simulink model "MSDR_v1"  (R2018a)
settings: Solver=ode23tb  StartTime=0.0  StopTime=50000  RelTol=1e-3
values from neighbouring files (symbols this model uses):
  a_f = -3.22E-5    (= -3.22e-05)    [MSDR_parameters.m]
  a_g = +2.35E-5    (= 2.35e-05)    [MSDR_parameters.m]
  beta = [0.000223, 0.001457, 0.001307, 0.002628, 0.000766, 0.000280]    [MSDR_parameters.m]
  beta_t = sum(beta)    [MSDR_parameters.m]
  Cp_s_shx = 1549.12e-6    (= 0.00154912)    [MSDR_parameters.m]
  Cst = 10    [MSDR_parameters.m]
  dLb = 0    [MSDR_parameters.m]
  dLs = 0    [MSDR_parameters.m]
  dLsc = 0    [MSDR_parameters.m]
  gamma_I = 5.1135e-2    (= 0.051135)    [MSDR_parameters.m]
  gamma_Xe = 1.1628e-2    (= 0.011628)    [MSDR_parameters.m]
  hA_fg = [h_fg*A_fg/2, h_fg*A_fg/2]    [MSDR_parameters.m]
  hA_p_phx1 = h_p_phx*A_p_phx    [MSDR_parameters.m]
  hA_p_phx2 = h_p_phx*A_p_phx    [MSDR_parameters.m]
  hA_p_phx3 = h_p_phx*A_p_phx    [MSDR_parameters.m]
  hA_p_phx4 = h_p_phx*A_p_phx    [MSDR_parameters.m]
  hA_p_phx5 = h_p_phx*A_p_phx    [MSDR_parameters.m]
  hA_p_phx6 = h_p_phx*A_p_phx    [MSDR_parameters.m]
  hA_p_shx1 = h_p_shx*A_p_shx    [MSDR_parameters.m]
  hA_p_shx2 = h_p_shx*A_p_shx    [MSDR_parameters.m]
  hA_p_shx3 = h_p_shx*A_p_shx    [MSDR_parameters.m]
  hA_p_shx4 = h_p_shx*A_p_shx    [MSDR_parameters.m]
  hA_p_shx5 = h_p_shx*A_p_shx    [MSDR_parameters.m]
  hA_p_shx6 = h_p_shx*A_p_shx    [MSDR_parameters.m]
  hA_s_phx1 = h_s_phx*A_s_phx    [MSDR_parameters.m]
  hA_s_phx2 = h_s_phx*A_s_phx    [MSDR_parameters.m]
  hA_s_phx3 = h_s_phx*A_s_phx    [MSDR_parameters.m]
  hA_s_phx4 = h_s_phx*A_s_phx    [MSDR_parameters.m]
  hA_s_phx5 = h_s_phx*A_s_phx    [MSDR_parameters.m]
  hA_s_phx6 = h_s_phx*A_s_phx    [MSDR_parameters.m]
  hA_s_shx1 = h_s_shx*A_s_shx    [MSDR_parameters.m]
  hA_s_shx2 = h_s_shx*A_s_shx    [MSDR_parameters.m]
  hA_s_shx3 = h_s_shx*A_s_shx    [MSDR_parameters.m]
  hA_s_shx4 = h_s_shx*A_s_shx    [MSDR_parameters.m]
  hA_s_shx5 = h_s_shx*A_s_shx    [MSDR_parameters.m]
  hA_s_shx6 = h_s_shx*A_s_shx    [MSDR_parameters.m]
  I_0 = gamma_I*Sig_f_msdr*phi_0/lam_I    (= 4.38204721773e+16)    [MSDR_parameters.m]
  Ifa = [0.25, 0.25]    [MSDR_parameters.m]
  Ifb = [0.25, 0.25]    [MSDR_parameters.m]
  Ig = [0.5, 0.5]    [MSDR_parameters.m]
  J = 1e-6    (= 1e-06)    [MSDR_parameters.m]
  ka = [0.235, 0.235]    [MSDR_parameters.m]
  kb = [0.235, 0.235]    [MSDR_parameters.m]
  kc = 5    [MSDR_parameters.m]
  kga = [0.015, 0.015]    [MSDR_parameters.m]
  kgb = [0.015, 0.015]    [MSDR_parameters.m]
  L = 8.5344    [MSDR_parameters.m]
  Lam = 2.400E-04    (= 0.00024)    [MSDR_parameters.m]
  lam = [0.0124, 0.0305, 0.111, 0.301, 1.14, 3.01]    [MSDR_parameters.m]
  lam_bubl = 2.0e-2    (= 0.02)    [MSDR_parameters.m]
  lam_I = 2.875e-5    (= 2.875e-05)    [MSDR_parameters.m]
  lam_Xe = 2.0916e-5    (= 2.0916e-05)    [MSDR_parameters.m]
  m_3m = W_3*2    (= 8618.207327)    [MSDR_parameters.m]
  m_fm = W_f*2    (= 9978.96)    [MSDR_parameters.m]
  m_sb = 1717    [MSDR_parameters.m]
  mb_cpb = 2.689619410657651e+00    (= 2.68961941066)    [MSDR_parameters.m]
  mcp_fa = mfa*Cp_f    [MSDR_parameters.m]
  mcp_fb = mfb*Cp_f    [MSDR_parameters.m]
  mcp_g = mg*Cp_g    [MSDR_parameters.m]
  mcp_p_phx1 = Cp_p_phx*mp_phx1    [MSDR_parameters.m]
  mcp_p_phx2 = Cp_p_phx*mp_phx2    [MSDR_parameters.m]
  mcp_p_phx3 = Cp_p_phx*mp_phx3    [MSDR_parameters.m]
  mcp_p_phx4 = Cp_p_phx*mp_phx4    [MSDR_parameters.m]
  mcp_p_phx5 = Cp_p_phx*mp_phx5    [MSDR_parameters.m]
  mcp_p_phx6 = Cp_p_phx*mp_phx6    [MSDR_parameters.m]
  mcp_p_shx1 = Cp_p_shx*mp_shx1    [MSDR_parameters.m]
  mcp_p_shx2 = Cp_p_shx*mp_shx2    [MSDR_parameters.m]
  mcp_p_shx3 = Cp_p_shx*mp_shx3    [MSDR_parameters.m]
  mcp_p_shx4 = Cp_p_shx*mp_shx4    [MSDR_parameters.m]
  mcp_p_shx5 = Cp_p_shx*mp_shx5    [MSDR_parameters.m]
  mcp_p_shx6 = Cp_p_shx*mp_shx6    [MSDR_parameters.m]
  mcp_s_phx1 = Cp_s_phx*ms_phx1    [MSDR_parameters.m]
  mcp_s_phx2 = Cp_s_phx*ms_phx2    [MSDR_parameters.m]
  mcp_s_phx3 = Cp_s_phx*ms_phx3    [MSDR_parameters.m]
  mcp_s_phx4 = Cp_s_phx*ms_phx4    [MSDR_parameters.m]
  mcp_s_phx5 = Cp_s_phx*ms_phx5    [MSDR_parameters.m]
  mcp_s_phx6 = Cp_s_phx*ms_phx6    [MSDR_parameters.m]
  mcp_s_shx1 = Cp_s_shx*ms_shx1    [MSDR_parameters.m]
  mcp_s_shx2 = Cp_s_shx*ms_shx1    [MSDR_parameters.m]
  mcp_s_shx3 = Cp_s_shx*ms_shx1    [MSDR_parameters.m]
  mcp_s_shx4 = Cp_s_shx*ms_shx1    [MSDR_parameters.m]
  mcp_s_shx5 = Cp_s_shx*ms_shx1    [MSDR_parameters.m]
  mcp_s_shx6 = Cp_s_shx*ms_shx1    [MSDR_parameters.m]
  mcp_t_phx1 = Cp_t_phx*mt_phx1    [MSDR_parameters.m]
  mcp_t_phx2 = Cp_t_phx*mt_phx2    [MSDR_parameters.m]
  mcp_t_phx3 = Cp_t_phx*mt_phx3    [MSDR_parameters.m]
  mcp_t_phx4 = Cp_t_phx*mt_phx4    [MSDR_parameters.m]
  mcp_t_phx5 = Cp_t_phx*mt_phx5    [MSDR_parameters.m]
  mcp_t_phx6 = Cp_t_phx*mt_phx6    [MSDR_parameters.m]
  mcp_t_shx1 = Cp_t_phx*mt_shx1    [MSDR_parameters.m]
  mcp_t_shx2 = Cp_t_phx*mt_shx2    [MSDR_parameters.m]
  mcp_t_shx3 = Cp_t_phx*mt_shx3    [MSDR_parameters.m]
  mcp_t_shx4 = Cp_t_phx*mt_shx4    [MSDR_parameters.m]
  mcp_t_shx5 = Cp_t_phx*mt_shx5    [MSDR_parameters.m]
  mcp_t_shx6 = Cp_t_phx*mt_shx6    [MSDR_parameters.m]
  mfa = [mass_fn, mass_fn]    [MSDR_parameters.m]
  mfb = [mass_fn, mass_fn]    [MSDR_parameters.m]
  mp_phx1 = [494.7, 494.7, 494.7, 494.7]    [MSDR_parameters.m]
  mp_phx2 = [494.7, 494.7, 494.7, 494.7]    [MSDR_parameters.m]
  mp_phx3 = [494.7, 494.7, 494.7, 494.7]    [MSDR_parameters.m]
  mp_phx4 = [494.7, 494.7, 494.7, 494.7]    [MSDR_parameters.m]
  mp_phx5 = [494.7, 494.7, 494.7, 494.7]    [MSDR_parameters.m]
  mp_phx6 = [494.7, 494.7, 494.7, 494.7]    [MSDR_parameters.m]
  mp_phxm = (Wp_phx1 + Wp_phx2)*1    (= 1663.16)    [MSDR_parameters.m]
  mp_shx1 = [429.3, 429.3, 429.3, 429.3]    [MSDR_parameters.m]
  mp_shx2 = [429.3, 429.3, 429.3, 429.3]    [MSDR_parameters.m]
  mp_shx3 = [429.3, 429.3, 429.3, 429.3]    [MSDR_parameters.m]
  mp_shx4 = [429.3, 429.3, 429.3, 429.3]    [MSDR_parameters.m]
  mp_shx5 = [429.3, 429.3, 429.3, 429.3]    [MSDR_parameters.m]
  mp_shx6 = [429.3, 429.3, 429.3, 429.3]    [MSDR_parameters.m]
  mp_shxm = (Wp_shx1 + Wp_shx2)*1    (= 932.38)    [MSDR_parameters.m]
  ms_phx1 = [1152.5, 1152.5, 1152.5, 1152.5]    [MSDR_parameters.m]
  ms_phx2 = [1152.5, 1152.5, 1152.5, 1152.5]    [MSDR_parameters.m]
  ms_phx3 = [1152.5, 1152.5, 1152.5, 1152.5]    [MSDR_parameters.m]
  ms_phx4 = [1152.5, 1152.5, 1152.5, 1152.5]    [MSDR_parameters.m]
  ms_phx5 = [1152.5, 1152.5, 1152.5, 1152.5]    [MSDR_parameters.m]
  ms_phx6 = [1152.5, 1152.5, 1152.5, 1152.5]    [MSDR_parameters.m]
  ms_phxm = (Ws_phx1 + Ws_phx2)*1    (= 932.38)    [MSDR_parameters.m]
  ms_shx1 = [1861.5, 1861.5, 1861.5, 1861.5]    [MSDR_parameters.m]
  ms_shx2 = [1861.5, 1861.5, 1861.5, 1861.5]    [MSDR_parameters.m]
  ... (+104 more)
undefined symbols (not defined in the file or in its folder): Ak2, As, C0, Cpp, Cps, Cpsc, Cpw, Dit, Dot, hA_p_thx1, hA_p_thx2, hA_p_thx3, hA_s_thx1, hA_s_thx2, hA_s_thx3, hc0, hfg, hfw0, HFW1, hfw10, HFW2, hpw, Hr, hr0, hwb, hws, hwsc, K3, KBHP, KBLP, Lsc, mcp_p_thx1, mcp_p_thx2, mcp_p_thx3, mcp_s_thx1, mcp_s_thx2, mcp_s_thx3, mcp_t_thx1, mcp_t_thx2, mcp_t_thx3, mp_thx1, mp_thx2, mp_thx3, ms_thx1, ms_thx2, ms_thx3, Mstm, nuf, Pp2, Pp3, Pp4, Pp5
libraries: simulink x20, aerolibconvert2 x2
(part 7 of 7)

== system MSDR_v1/BALANCE OF PLANT/POWER/BOP/Nozzle Chest ==
  note: 843-0.4*(u[13]-200)
  note: 3.353614E-26*u(13)^6 - 9.257963E-21*u(13)^5 + 9.864059E-16*u(13)^4 - 5.121756E-11*u(13)^3 + 1.364869E-06*u(13)^2 - 2.062660E-02*u(13) + 1.016796E+03
  note: -4.63411E-18*u(13)^4 + 1.20033E-12*u(13)^3 - 1.23684E-07*u(13)^2 + 7.74471E-03*u(13) + 2.09721E+02
  note: 3.16015E-28*u(13)^6 - 1.06919E-22*u(13)^5 + 1.47784E-17*u(13)^4 - 1.07591E-12*u(13)^3 + 4.43489E-08*u(13)^2 - 1.03385E-03*u(13) + 1.27494E+01
  note: ((w1*hs-w2*hc)/rhoc*Vc)+(J*Pc/rhoc^2)*drhoc/dt)
  note: (u[16]-u[11])*(u[12])
  note: 1/(u[8]*u[10]+(1-u[8])*nuf)
  note: Ak2*(u[7]*u[4]-u[13]*u[9])^.5
  note: (((u[15]*u[14]-u[6]*u[2])*u[5]/VC)+(J*u[7]*u[5]^2*u[3]))
  note: (u[15]-u[6])/VC
  note: Ak2*(Pc*rhoc-Pr*rho2)
  note: (w1-w2)/Vc
  note: (h2-hf)/hfg
  note: 1/(x*nug+(1-x)*nuf)
  w1 : Inport
  hs : Inport  Port=2
  h2 : Inport  Port=3
  PR : Inport  Port=4
  1/hfg : Math  Operator=reciprocal  SaturateOnIntegerOverflow=on
  1/rhoc : Math  Operator=reciprocal  SaturateOnIntegerOverflow=on
  Display1 : Display
  Display15 : Display
      settings: Format=decimal (Stored Integer)
  Init2 : InitialCondition  Value=1/hfg
  Mux1 : Mux  Inputs=16
      settings: DisplayOption=signals
  PC 2-D Lookup Table : Lookup_n-D  BreakpointsForDimension1=[800,810.204081632653,820.408163265306,830.612244897959,840.816326530612,851.020408163265,861.224489795918,871.428571428571,881.632653061225,891.836734693878,902.040816326531,912.244897959184,922.448979591837,932.653061224490,942.857142857143,953.061224489796,963.265306122449,973.469387755102,983.673469387755,993.877551020408,1004.08163265306,1014.28571428571,1024.48979591837,1034.69387755102,1044.89795918367,1055.10204081633,1065.30612244898,1075.51020408163,1085.71428571429,1095.91836734694,1106.12244897959,1116.32653061224,1126.53061224490,1136.73469387755,1146.93877551020,1157.14285714286,1167.34693877551,1177.55102040816,1187.75510204082,1197.95918367347,1208.16326530612,1218.36734693878,1228.57142857143,1238.77551020408,1248.97959183673,1259.18367346939,1269.38775510204,1279.59183673469,1289.79591836735,1300]  BreakpointsForDimension2=[0.7000,1.0000,1.300,1.6000,1.9000 ,2.2000]  Table=|  InternalRulePriority=Speed  RndMeth=Simplest  InputSameDT=on
      | [0.1716    0.2398    0.3051    0.3680    0.4286    0.4872;    0.1752    0.2450    0.3120    0.3765    0.4387    0.4989
      | ;    0.1788    0.2502    0.3189    0.3850    0.4489    0.5107
      | ;    0.1824    0.2555    0.3258    0.3936    0.4591    0.5226
      | ;    0.1861    0.2608    0.3327    0.4022    0.4694    0.5345
      | ;    0.1897    0.2661    0.3398    0.4109    0.4797    0.5465
      | ;    0.1934    0.2715    0.3468    0.4196    0.4902    0.5586
      | ;    0.1971    0.2768    0.3539    0.4284    0.5006    0.5708
      | ;    0.2008    0.2822    0.3610    0.4372    0.5111    0.5830
      | ;    0.2045    0.2877    0.3681    0.4461    0.5217    0.5952
      | ;    0.2082    0.2931    0.3753    0.4550    0.5324    0.6076
      | ;    0.2120    0.2986    0.3825    0.4639    0.5430    0.6200
      | ;    0.2157    0.3041    0.3897    0.4729    0.5538    0.6325
      | ;    0.2195    0.3096    0.3970    0.4820    0.5646    0.6450
      | ;    0.2233    0.3151    0.4043    0.4910    0.5754    0.6576
      | ;    0.2271    0.3207    0.4117    0.5001    0.5863    0.6703
      | ;    0.2309    0.3263    0.4190    0.5093    0.5972    0.6830
      | ;    0.2347    0.3319    0.4264    0.5185    0.6082    0.6958
      | ;    0.2386    0.3375    0.4339    0.5277    0.6193    0.7086
      | ;    0.2424    0.3432    0.4413    0.5370    0.6304    0.7215
      | ;    0.2463    0.3488    0.4488    0.5463    0.6415    0.7344
      | ;    0.2502    0.3545    0.4563    0.5557    0.6527    0.7474
      | ;    0.2541    0.3602    0.4639    0.5650    0.6639    0.7605
      | ;    0.2580    0.3660    0.4714    0.5745    0.6751    0.7736
      | ;    0.2619    0.3717    0.4790    0.5839    0.6865    0.7867
      | ;    0.2659    0.3775    0.4867    0.5934    0.6978    0.7999
      | ;    0.2698    0.3833    0.4943    0.6029    0.7092    0.8132
      | ;    0.2738    0.3891    0.5020    0.6125    0.7206    0.8265
      | ;    0.2777    0.3949    0.5097    0.6221    0.7321    0.8398
      | ;    0.2817    0.4008    0.5174    0.6317    0.7436    0.8532
      | ;    0.2857    0.4066    0.5252    0.6414    0.7552    0.8667
      | ;    0.2897    0.4125    0.5330    0.6511    0.7668    0.8802
      | ;    0.2937    0.4184    0.5408    0.6608    0.7784    0.8937
      | ;    0.2978    0.4243    0.5486    0.6705    0.7901    0.9073
      | ;    0.3018    0.4303    0.5565    0.6803    0.8018    0.9209
      | ;    0.3059    0.4362    0.5643    0.6901    0.8135    0.9346
      | ;    0.3099    0.4422    0.5722    0.7000    0.8253    0.9483
      | ;    0.3140    0.4482    0.5802    0.7098    0.8371    0.9620
      | ;    0.3181    0.4542    0.5881    0.7197    0.8490    0.9758
      | ;    0.3222    0.4602    0.5961    0.7296    0.8614    0.9953
      | ;    0.3281    0.4680    0.6072    0.7459    0.8839    1.0215
      | ;    0.3366    0.4801    0.6230    0.7652    0.9069    1.0480
      | ;    0.3454    0.4924    0.6389    0.7847    0.9301    1.0749
      | ;    0.3541    0.5049    0.6550    0.8045    0.9534    1.1019
      | ;    0.3630    0.5174    0.6711    0.8243    0.9769    1.1291
      | ;    0.3718    0.5299    0.6874    0.8442    1.0005    1.1564
      | ;    0.3807    0.5425    0.7037    0.8642    1.0242    1.1838
      | ;    0.3895    0.5551    0.7200    0.8843    1.0480    1.2113
      | ;    0.3984    0.5678    0.7364    0.9044    1.0719    1.2389
      | ;    0.4073    0.5804    0.7528    0.9246    1.0958    1.2666
      | ]
  dhc/dt : Fcn  Expr=(((u[15]*u[14]-u[6]*u[2])*u[5]/VC)+(J*u[7]*u[5]^2*u[3]))
  drhoc/dt : Fcn  Expr=(u[15]-u[6])/VC
  hc_in : Fcn  Expr=u(2)
  hc_out : Integrator  InitialCondition=hc0
  hf : Fcn  Expr=-4.63411E-18*u(13)^4 + 1.20033E-12*u(13)^3 - 1.23684E-07*u(13)^2 + 7.74471E-03*u(13) + 2.09721E+02
  hfg : Fcn  Expr=3.353614E-26*u(13)^6 - 9.257963E-21*u(13)^5 + 9.864059E-16*u(13)^4 - 5.121756E-11*u(13)^3 + 1.364869E-06*u(13)^2 - 2.062660E-02*u(13) + 1.016796E+03
  hfg1 : Fcn  Expr=843-0.4*(u[13]/144-200)
  nug : Fcn  Expr=3.16015E-28*u(13)^6 - 1.06919E-22*u(13)^5 + 1.47784E-17*u(13)^4 - 1.07591E-12*u(13)^3 + 4.43489E-08*u(13)^2 - 1.03385E-03*u(13) + 1.27494E+01
  output : ToWorkspace  VariableName=cst  SampleTime=-1
  "psi -> psf" : Gain  Gain=1000*144
  rho2 : Fcn  Expr=1/(u[8]*u[10]+(1-u[8])*nuf)
  rhoc : Integrator  InitialCondition=rhoc0
  rhoc_in : Fcn  Expr=u(4)
  scope1 : Scope
  scope2 : Scope
  scope4 : Scope
  w2_out : Fcn  Expr=Ak2*(u[7]*u[4]-u[13]*u[9])^.5
  x : Fcn  Expr=(u[16]-u[11])*(u[12])
  hfg_out : Outport
  hf_out : Outport  Port=2
  w2 : Outport  Port=3
  hc : Outport  Port=4
  PC : Outport  Port=5
  wires:
  drhoc/dt/1 -> Mux1/3, rhoc/1
  w2_out/1 -> w2/1, Mux1/6
  rhoc/1 -> Mux1/4, 1/rhoc/1
  hc_out/1 -> hc/1, Mux1/2
  dhc/dt/1 -> Mux1/1, hc_out/1
  nug/1 -> Mux1/10
  hf/1 -> scope1/1, hf_out/1, Mux1/11
  1/hfg/1 -> Init2/1
  1/rhoc/1 -> Mux1/5
  PR/1 -> Mux1/13
  rho2/1 -> scope2/1, Mux1/9
  hs/1 -> Mux1/14
  w1/1 -> Mux1/15
  h2/1 -> Mux1/16
  x/1 -> Mux1/8
  rhoc_in/1 -> PC 2-D Lookup Table/2
  hc_in/1 -> PC 2-D Lookup Table/1
  PC 2-D Lookup Table/1 -> "psi -> psf"/1
  "psi -> psf"/1 -> PC/1, Mux1/7
  Mux1/1 -> hfg1/1, hfg/1, hf/1, nug/1, rho2/1, x/1, w2_out/1, drhoc/dt/1, dhc/dt/1, hc_in/1, rhoc_in/1, output/1
  hfg/1 -> Display1/1, 1/hfg/1, hfg_out/1, scope4/1
  Init2/1 -> Mux1/12
  hfg1/1 -> Display15/1

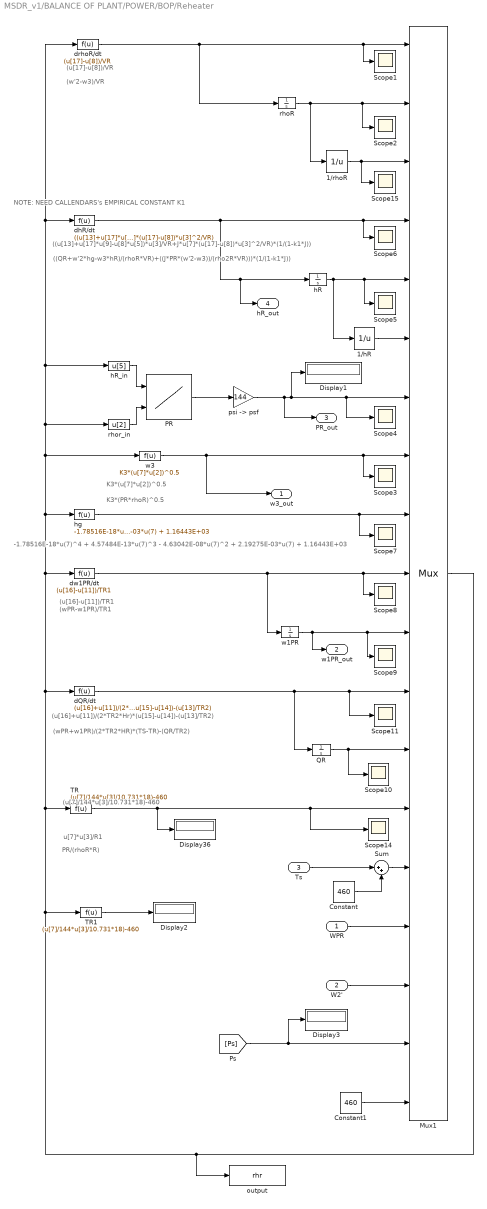
== system MSDR_v1/BALANCE OF PLANT/POWER/BOP/Reheater ==
  note: (u[7]/144*u[3]/10.731*18)-460
  note: NOTE: NEED CALLENDARS's EMPIRICAL CONSTANT K1
  note: -1.78516E-18*u(7)^4 + 4.57484E-13*u(7)^3 - 4.63042E-08*u(7)^2 + 2.19275E-03*u(7) + 1.16443E+03
  note: (wPR+w1PR)/(2*TR2*HR)*(TS-TR)-(QR/TR2)
  note: (u[16]+u[11])/(2*TR2*Hr)*(u[15]-u[14])-(u[13]/TR2)
  note: u[7]*u[3]/R1
  note: K3*(u[7]*u[2])^0.5
  note: (u[17]-u[8])/VR
  note: (wPR-w1PR)/TR1
  note: K3*(PR*rhoR)^0.5
  note: ((QR+w'2*hg-w3*hR)/(rhoR*VR)+((J*PR*(w'2-w3))/(rho2R*VR)))*(1/(1-k1*J))
  note: (w'2-w3)/VR
  note: (u[16]-u[11])/TR1
  note: PR/(rhoR*R)
  note: ((u[13]+u[17]*u[9]-u[8]*u[5])*u[3]/VR+J*u[7]*(u[17]-u[8])*u[3]^2/VR)*(1/(1-k1*J))
  WPR : Inport
  W2' : Inport  Port=2
  Ts : Inport  Port=3
  1/hR : Math  Operator=reciprocal  SaturateOnIntegerOverflow=on
  1/rhoR : Math  Operator=reciprocal  SaturateOnIntegerOverflow=on
  Constant : Constant  Value=460
  Constant1 : Constant  Value=460
  Display{1..3,36} (4 alike) : Display
  Mux1 : Mux  Inputs=19
      settings: DisplayOption=signals
  PR : Lookup_n-D  BreakpointsForDimension1=[800,826.315789473684,852.631578947368,878.947368421053,905.263157894737,931.578947368421,957.894736842105,984.210526315790,1010.52631578947,1036.84210526316,1063.15789473684,1089.47368421053,1115.78947368421,1142.10526315789,1168.42105263158,1194.73684210526,1221.05263157895,1247.36842105263,1273.68421052632,1300]  BreakpointsForDimension2=[0.1,0.2,0.3,0.4,0.5,0.6]  Table=[25.3463,50.7407,75.7363,100.3099,124.4733,148.2447;26.4874,53.1606,79.4857,105.4185,130.9601,156.1229;27.6372,55.6021,83.2719,110.5805,137.5187,164.0922;28.7954,58.0643,87.0934,115.7941,144.1462,172.1489;29.9618,60.5467,90.9489,121.0572,150.84,180.2899;31.1361,63.0485,94.8374,126.3682,157.5979,188.512;32.318,65.5689,98.7576,131.7255,164.4176,196.8124;33.5074,68.1076,102.7086,137.1274,171.297,205.1885;34.704,70.6639,106.6893,142.5726,178.2341,213.6376;35.9075,73.2372,110.699,148.0597,185.2271,222.1574;37.1178,75.8272,114.7367,153.5874,192.2744,230.7457;38.3347,78.4333,118.8016,159.1546,199.3741,239.4004;39.5581,81.0551,122.893,164.7601,206.5249,248.1194;40.7877,83.6922,127.0101,170.4029,213.7253,256.901;42.0235,86.3442,131.1523,176.0819,220.9739,265.7434;45.1641,90.4145,135.7246,181.7961,228.2693,274.6447;48.5193,97.0218,145.4961,193.9318,242.3206,290.6561;51.8711,103.6672,155.3921,207.046,258.6271,310.1328;55.2084,110.3074,165.3066,220.2121,275.0271,329.7535;58.5245,116.9217,175.2023,233.3741,291.4438,349.4156]  InternalRulePriority=Speed  RndMeth=Simplest  InputSameDT=on
  QR : Integrator  InitialCondition=QR0
  Scope{1..11,14..15} (13 alike) : Scope
  Sum : Sum  Inputs=|++
  TR : Fcn  Expr=(u[7]/144*u[3]/10.731*18)-460
  TR1 : Fcn  Expr=(u[7]/144*u[3]/10.731*18)-460
  dQR/dt : Fcn  Expr=(u[16]+u[11])/(2*TR2*Hr)*(u[15]-u[14])-(u[13]/TR2)
  dhR/dt : Fcn  Expr=((u[13]+u[17]*u[9]-u[8]*u[5])*u[3]/VR+J*u[7]*(u[17]-u[8])*u[3]^2/VR)
  drhoR/dt : Fcn  Expr=(u[17]-u[8])/VR
  dw1PR/dt : Fcn  Expr=(u[16]-u[11])/TR1
  hR : Integrator  InitialCondition=hr0
  hR_in : Fcn  Expr=u[5]
  hg : Fcn  Expr=-1.78516E-18*u(7)^4 + 4.57484E-13*u(7)^3 - 4.63042E-08*u(7)^2 + 2.19275E-03*u(7) + 1.16443E+03
  output : ToWorkspace  VariableName=rhr  SampleTime=-1
  "psi -> psf" : Gain  Gain=144
  rhoR : Integrator  InitialCondition=rhor0
  rhor_in : Fcn  Expr=u[2]
  w1PR : Integrator  InitialCondition=wpr10
  w3 : Fcn  Expr=K3*(u[7]*u[2])^0.5
  w3_out : Outport
  w1PR_out : Outport  Port=2
  PR_out : Outport  Port=3
  hR_out : Outport  Port=4
  wires:
  drhoR/dt/1 -> Scope1/1, Mux1/1, rhoR/1
  dhR/dt/1 -> Mux1/4, Scope6/1, hR_out/1, hR/1
  rhoR/1 -> Scope2/1, Mux1/2, 1/rhoR/1
  hR/1 -> 1/hR/1, Mux1/5, Scope5/1
  w3/1 -> Mux1/8, Scope3/1, w3_out/1
  hg/1 -> Mux1/9, Scope7/1
  dw1PR/dt/1 -> Mux1/10, Scope8/1, w1PR/1
  w1PR/1 -> Mux1/11, Scope9/1, w1PR_out/1
  dQR/dt/1 -> Mux1/12, Scope11/1, QR/1
  QR/1 -> Mux1/13, Scope10/1
  WPR/1 -> Mux1/16
  W2'/1 -> Mux1/17
  1/rhoR/1 -> Mux1/3, Scope15/1
  1/hR/1 -> Mux1/6
  Ts/1 -> Sum/1
  Constant/1 -> Sum/2
  Sum/1 -> Mux1/15
  TR/1 -> Display36/1, Mux1/14, Scope14/1
  hR_in/1 -> PR/1
  rhor_in/1 -> PR/2
  PR/1 -> "psi -> psf"/1
  "psi -> psf"/1 -> PR_out/1, Display1/1, Scope4/1, Mux1/7
  Mux1/1 -> TR1/1, w3/1, rhor_in/1, drhoR/dt/1, dhR/dt/1, hR_in/1, hg/1, dw1PR/dt/1, dQR/dt/1, TR/1, output/1
  TR1/1 -> Display2/1
  [Ps] -> Display3/1, Mux1/18
  Constant1/1 -> Mux1/19

== system MSDR_v1/BALANCE OF PLANT/POWER/BOP/Secondary Steam Valve ==
  Ws : Inport
  Product : Product
  SSV Coefficient : Constant  Value=.16
  output : ToWorkspace  VariableName=wpr  SampleTime=-1
  WPR : Outport
  wires:
  Ws/1 -> Product/2
  Product/1 -> WPR/1, output/1
  SSV Coefficient/1 -> Product/1

== system MSDR_v1/HEAT EXCHANGERS/HEAT EXCHANGER LOOP 1/Fractional Power Demand (fractional)/Slider ==

== system MSDR_v1/HEAT EXCHANGERS/HEAT EXCHANGER LOOP 2/Fractional Power Demand (fractional)/Slider ==

== system MSDR_v1/HEAT EXCHANGERS/HEAT EXCHANGER LOOP 3/Fractional Power Demand (fractional)/Slider ==

== system MSDR_v1/HEAT EXCHANGERS/HEAT EXCHANGER LOOP 4/Fractional Power Demand (fractional)/Slider ==

== system MSDR_v1/HEAT EXCHANGERS/HEAT EXCHANGER LOOP 5/Fractional Power Demand (fractional)/Slider ==

== system MSDR_v1/HEAT EXCHANGERS/HEAT EXCHANGER LOOP 6/Fractional Power Demand (fractional)/Slider ==
